simulink model "Thrust_Inclination"  (R2016b)
settings: Solver=FixedStepAuto  StartTime=0.0  StopTime=tf  FixedStep=0.01  RelTol=1e-3
values from neighbouring files (symbols this model uses):
  D_rho = 5*10    (= 50)    [P_1.m]    (also in P_10_Optimal.m; P_15_rt_tgo.m; P_9_tgo_dlmbda.m)
  R0 = eq2(t_1)    [P_1.m]
  rx_0 = r0*cos(lmbda_0)    [P_1.m]    (also in P_9_tgo_dlmbda.m)
  ry_0 = r0*sin(lmbda_0)    [P_1.m]    (also in P_9_tgo_dlmbda.m)
  Vc = r_norm./tgo_int    [Nir_ref.m]
undefined symbols (not defined in the file or in its folder): drx_0, dry_0, K, K_dth, M_d, T_m
settings Model: Creator=Daniel  LastModifiedBy=Daniel

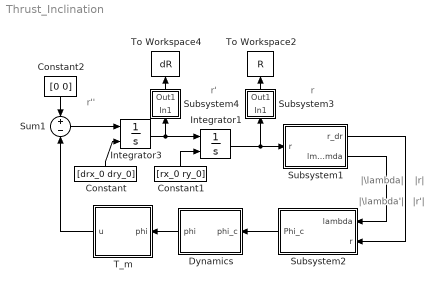
== system Thrust_Inclination ==
  note: r'
  note: r
  note: r''
  note: |r|
  note: |r'|
  note: |\lambda|
  note: |\lambda'|
  Constant : Constant  Value=[drx_0 dry_0]
  Constant1 : Constant  Value=[rx_0 ry_0]
  Constant2 : Constant  Value=[0 0]
  Dynamics : Subsystem
      mask Display: image('12_AP.PNG');
  Integrator1 : Integrator  InitialConditionSource=external  InitialCondition=Vc
  Integrator3 : Integrator  InitialConditionSource=external  InitialCondition=R0
  Subsystem1 : Subsystem
      mask Display: image('12_geometry.PNG');
  Subsystem2 : Subsystem
      mask Display: image('12_Phi.PNG');
  Subsystem3 : Subsystem
      mask Display: image('norm.PNG');
  Subsystem4 : Subsystem
      mask Display: image('norm.PNG');
  Sum1 : Sum  Inputs=+|-
  T_m : Subsystem
      mask Display: image('12_T_m.PNG');
  To Workspace2 : ToWorkspace  VariableName=R  SaveFormat=Timeseries  SampleTime=-1
  To Workspace4 : ToWorkspace  VariableName=dR  SaveFormat=Timeseries  SampleTime=-1
  wires:
  Constant1/1 -> Integrator1/2
  Constant/1 -> Integrator3/2
  Dynamics/1(phi) -> T_m/1(phi)
  T_m/1(u) -> Sum1/2
  Sum1/1 -> Integrator3/1
  Constant2/1 -> Sum1/1
  Subsystem1/2(lmda_dlmda) -> Subsystem2/1(lambda)
  Subsystem1/1(r_dr) -> Subsystem2/2(r)
  Subsystem2/1(Phi_c) -> Dynamics/1(phi_c)
  Subsystem4/1(Out1) -> To Workspace4/1
  Integrator1/1 -> Subsystem1/1(r), Subsystem3/1(In1)
  Subsystem3/1(Out1) -> To Workspace2/1
  Integrator3/1 -> Subsystem4/1(In1), Integrator1/1

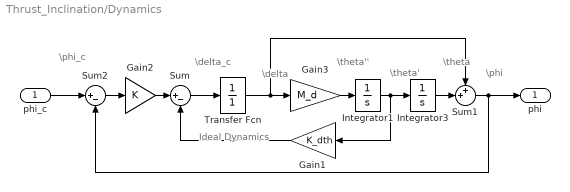
== system Thrust_Inclination/Dynamics ==
  note: Ideal Dynamics
  note: \theta'
  note: \theta''
  note: \theta
  note: \delta
  note: \delta_c
  note: \phi_c
  note: \phi
  phi_c : Inport
  Gain1 : Gain  Gain=K_dth
  Gain2 : Gain  Gain=K
  Gain3 : Gain  Gain=M_d
  Integrator1 : Integrator
  Integrator3 : Integrator
  Sum : Sum  Inputs=|+-
  Sum1 : Sum  Inputs=++|
  Sum2 : Sum  Inputs=|+-
  Transfer Fcn : TransferFcn  Denominator=[0 1]
  phi : Outport
  wires:
  Gain1/1 -> Sum/2
  Sum/1 -> Transfer Fcn/1
  Gain2/1 -> Sum/1
  Transfer Fcn/1 -> Sum1/1, Gain3/1
  Gain3/1 -> Integrator1/1
  Integrator1/1 -> Integrator3/1, Gain1/1
  Integrator3/1 -> Sum1/2
  Sum2/1 -> Gain2/1
  Sum1/1 -> phi/1, Sum2/2
  phi_c/1 -> Sum2/1

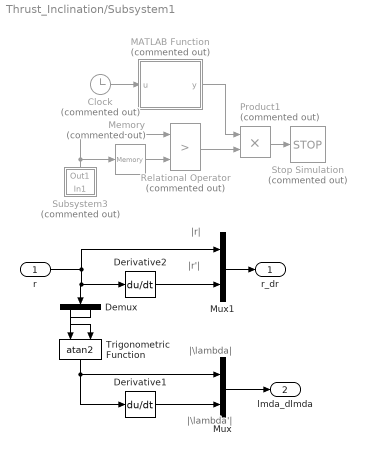
== system Thrust_Inclination/Subsystem1 ==
  note: |r|
  note: |r'|
  note: |\lambda|
  note: |\lambda'|
  r : Inport
  Clock : Clock  Commented=on
  Demux : Demux  Outputs=2
  Derivative1 : Derivative
  Derivative2 : Derivative
  MATLAB Function : MATLAB Function  Commented=on  TreatAsAtomicUnit=on
  Memory : Memory  Commented=on  InheritSampleTime=on
  Mux : Mux  Inputs=2
  Mux1 : Mux  Inputs=2
  Product1 : Product  Commented=on
  Relational Operator : RelationalOperator  Commented=on  Operator=>  OutDataTypeStr=boolean  RndMeth=Simplest
  Stop Simulation : Stop  Commented=on
  Subsystem3 : Subsystem  Commented=on
      mask Display: image('norm.PNG');
  Trigonometric Function : Trigonometry  Operator=atan2
  r_dr : Outport
  lmda_dlmda : Outport  Port=2
  wires:
  Derivative2/1 -> Mux1/2
  Trigonometric Function/1 -> Derivative1/1, Mux/1
  Mux1/1 -> r_dr/1
  Demux/1 -> Trigonometric Function/2
  Demux/2 -> Trigonometric Function/1
  Derivative1/1 -> Mux/2
  Mux/1 -> lmda_dlmda/1
  r/1 -> Mux1/1, Derivative2/1, Demux/1
  Memory/1 -> Relational Operator/2
  Subsystem3/1(Out1) -> Relational Operator/1, Memory/1
  Clock/1 -> MATLAB Function/1(u)
  Relational Operator/1 -> Product1/2
  MATLAB Function/1(y) -> Product1/1
  Product1/1 -> Stop Simulation/1

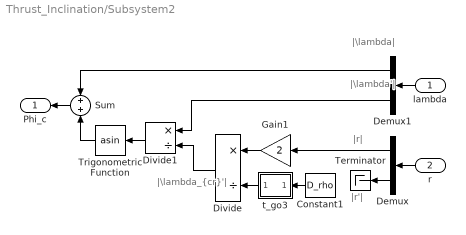
== system Thrust_Inclination/Subsystem2 ==
  note: |\lambda'|
  note: |\lambda|
  note: |r'|
  note: |r|
  note: |\lambda_{cr}'|
  lambda : Inport
  r : Inport  Port=2
  Constant1 : Constant  Value=D_rho
  Demux : Demux  Outputs=2
  Demux1 : Demux  Outputs=2
  Divide : Product  Inputs=*/
  Divide1 : Product  Inputs=*/
  Gain1 : Gain  Gain=2
  Sum : Sum  Inputs=+|+
  Terminator : Terminator
  Trigonometric Function : Trigonometry  Operator=asin
  t_go3 : Subsystem
      mask Display: image('t_go_P.PNG');
  Phi_c : Outport
  wires:
  r/1 -> Demux/1
  lambda/1 -> Demux1/1
  Constant1/1 -> t_go3/1(In1)
  Gain1/1 -> Divide/1
  Divide/1 -> Divide1/2
  Demux1/2 -> Divide1/1
  Trigonometric Function/1 -> Sum/2
  Demux1/1 -> Sum/1
  Sum/1 -> Phi_c/1
  Demux/1 -> Gain1/1
  Demux/2 -> Terminator/1
  Divide1/1 -> Trigonometric Function/1
  t_go3/1(Out1) -> Divide/2

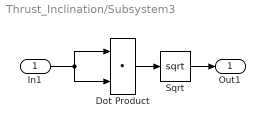
== system Thrust_Inclination/Subsystem3 ==
  In1 : Inport
  Dot Product : DotProduct  InputSameDT=on  OutDataTypeStr=Inherit: Inherit via internal rule
  Sqrt : Sqrt  SaturateOnIntegerOverflow=on
  Out1 : Outport
  wires:
  Sqrt/1 -> Out1/1
  Dot Product/1 -> Sqrt/1
  In1/1 -> Dot Product/2, Dot Product/1

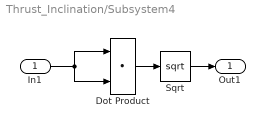
== system Thrust_Inclination/Subsystem4 ==
  In1 : Inport
  Dot Product : DotProduct  InputSameDT=on  OutDataTypeStr=Inherit: Inherit via internal rule
  Sqrt : Sqrt  SaturateOnIntegerOverflow=on
  Out1 : Outport
  wires:
  Sqrt/1 -> Out1/1
  Dot Product/1 -> Sqrt/1
  In1/1 -> Dot Product/2, Dot Product/1

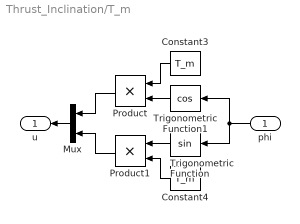
== system Thrust_Inclination/T_m ==
  phi : Inport
  Constant3 : Constant  Value=T_m
  Constant4 : Constant  Value=T_m
  Mux : Mux  Inputs=2
  Product : Product
  Product1 : Product
  Trigonometric Function : Trigonometry
  Trigonometric Function1 : Trigonometry  Operator=cos
  u : Outport
  wires:
  Trigonometric Function/1 -> Product1/1
  phi/1 -> Trigonometric Function/1, Trigonometric Function1/1
  Constant3/1 -> Product/1
  Constant4/1 -> Product1/2
  Product1/1 -> Mux/2
  Trigonometric Function1/1 -> Product/2
  Mux/1 -> u/1
  Product/1 -> Mux/1

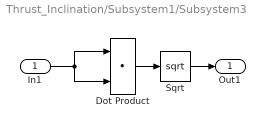
== system Thrust_Inclination/Subsystem1/Subsystem3 ==
  In1 : Inport
  Dot Product : DotProduct  InputSameDT=on  OutDataTypeStr=Inherit: Inherit via internal rule
  Sqrt : Sqrt  SaturateOnIntegerOverflow=on
  Out1 : Outport
  wires:
  Sqrt/1 -> Out1/1
  Dot Product/1 -> Sqrt/1
  In1/1 -> Dot Product/2, Dot Product/1

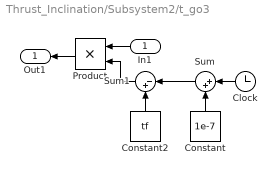
== system Thrust_Inclination/Subsystem2/t_go3 ==
  In1 : Inport
  Clock : Clock
  Constant : Constant  Value=1e-7
  Constant2 : Constant  Value=tf
  Product : Product
  Sum : Sum  Inputs=|++
  Sum1 : Sum  Inputs=|-+
  Out1 : Outport
  wires:
  Sum/1 -> Sum1/1
  Clock/1 -> Sum/1
  Sum1/1 -> Product/2
  Constant/1 -> Sum/2
  Constant2/1 -> Sum1/2
  In1/1 -> Product/1
  Product/1 -> Out1/1

== matlab function Thrust_Inclination/Subsystem1/MATLAB Function ==
  data: u input; y output
function y = fcn(u)
if u < 0.01
    y = 0;
else
    y = 1;
end
end
